simulink model "Pendulum"  (Simulink 5.0)
settings: Solver=ode45  StartTime=0.0  StopTime=inf  RelTol=1e-12  AbsTol=1e-9
values from neighbouring files (symbols this model uses):
  N = Nu + K*Nx    [PENDULUM.M]
libraries: mblibv1 x8
settings Model: LastModifiedBy=Administrator  BooleanDataType=off

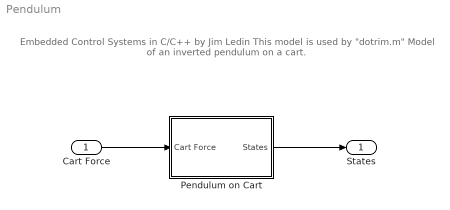
== system Pendulum ==
  note: Embedded Control Systems in C/C++
      | by Jim Ledin
      |
      | This model is used by "dotrim.m"
      |
      | Model of an inverted pendulum on a cart.
  Cart Force : Inport  PortDimensions=1
  Pendulum on Cart : Subsystem
  States : Outport
  wires:
  Cart Force/1 -> Pendulum on Cart/1(Cart Force)
  Pendulum on Cart/1(States) -> States/1

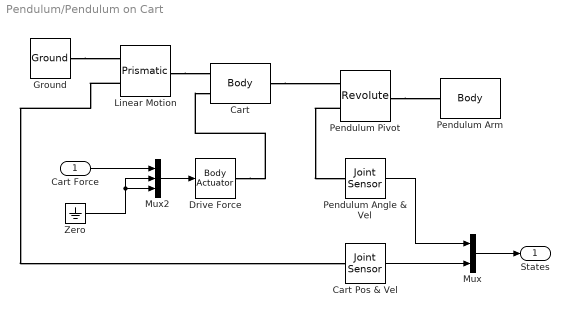
== system Pendulum/Pendulum on Cart ==
  Cart Force : Inport  PortDimensions=1
  Cart : mblibv1/Bodies/Body  Tag=Factory generic  Description=Mechanical Blockset  PhysicalDomain=mechanical  SubClassName=Unknown  PortType=workingframe  LConnTagsString=CS1|CG  RConnTagsString=CS2  DialogClass=MechanicalBodyBlock  Mass=5  MassUnits=kg  InertiaUnits=kg*m^2  Inertia=eye(3)  Shape=Cylinder  ShapeDims=[1 1]  ShapeUnits=m  ShapeUse=false  Density=1  DensityUnits=kg/m^3  DensityUse=false  CG=Left$CG$[0 0 0]$WORLD$WORLD$m$[0 0 0]$Euler X-Y-Z$deg$WORLD$true  WorkingFrames=Left$CS1$[0 0 0]$CG$CG$m$[0 0 0]$Euler X-Y-Z$deg$WORLD$true#Right$CS2$[0 0 0]$CG$CG$m$[0 0 0]$Euler X-Y-Z$deg$WORLD$true
  Cart Pos & Vel : mblibv1/Sensors &  Actuators/Joint Sensor  Tag=__orphan__  Description=Mechanical Blockset  PortType=blob  PhysicalDomain=Mechanical  Muxed=on  Pose=off  Angle=on  AngleUnits=deg  ArcVelocity=off  ArcVelocityUnits=deg/s  ArcAcceleration=off  ArcAccelerationUnits=deg/s²  CoordPosition=on  CoordPositionUnits=m  Velocity=on  VelocityUnits=m/s  Acceleration=off  AccelerationUnits=m/s²  Quaternion=on  QuaternionDT=off  QuaternionDDT=off  QuaternionUnits=off  OutputVector=[ 1 1 ]  ActiveIO=off  Width=1  DialogClass=MechanicalSensorBlock  Primitive=P1  Force=off  ForceUnits=N  Torque=off  TorqueUnits=N-m  ReferenceFrame=Absolute (INERTIAL)  ReactionSensedSide=Base  ReactionReferenceFrame=Absolute (World)  ReactionForce=off  ReactionForceUnits=N  ReactionMoment=off  ReactionMomentUnits=N-m
  Drive Force : mblibv1/Sensors &  Actuators/Body Actuator  Tag=__orphan__  Description=Mechanical Blockset  PortType=blob  PhysicalDomain=Mechanical  ActuationStyle=Force  AngleUnits=deg  ArcVelocityUnits=deg/s  ArcAccelerationUnits=deg/s^2  CoordPositionUnits=m  VelocityUnits=m/s  AccelerationUnits=m/s^2  ForceUnits=N  TorqueUnits=N-m  ActiveIO=off  Width=1  DialogClass=MechanicalActuatorBlock  ReferenceFrame=Absolute (INERTIAL)  Angle=off  CoordPosition=on  Force=on  Torque=off
  Ground : mblibv1/Bodies/Ground  Tag=__orphan__  PortType=workingframe  PhysicalDomain=Mechanical  DialogClass=GroundBlock  CoordPosition=[0 0 0]  CoordPositionUnits=m  StateVectorMgrId=-1  MachineId=[0 0]
  Linear Motion : mblibv1/Joints/Prismatic  Tag=Factory generic  Description=Mechanical Blockset  PhysicalDomain=mechanical  SubClassName=Unknown  PortType=blob  LConnTagsString=__newl0|SA1  RConnTagsString=__newr0  NumSAPorts=1  CutJoint=off  MarkAsCut=off  Primitives=prismatic  PrimitiveProps=P1$WORLD$[1 0 0]$prismatic  DialogClass=JointBlock
  Mux : Mux  Inputs=2
  Mux2 : Mux  Inputs=3
  Pendulum Angle & Vel : mblibv1/Sensors &  Actuators/Joint Sensor  Tag=__orphan__  Description=Mechanical Blockset  PortType=blob  PhysicalDomain=Mechanical  Muxed=on  Pose=off  Angle=on  AngleUnits=rad  ArcVelocity=on  ArcVelocityUnits=rad/s  ArcAcceleration=off  ArcAccelerationUnits=deg/s^2  CoordPosition=on  CoordPositionUnits=m  Velocity=off  VelocityUnits=m/s  Acceleration=off  AccelerationUnits=m/s^2  Quaternion=on  QuaternionDT=off  QuaternionDDT=off  QuaternionUnits=off  OutputVector=[ 1 1 ]  ActiveIO=off  Width=1  DialogClass=MechanicalSensorBlock  Primitive=R1  Force=off  ForceUnits=N  Torque=off  TorqueUnits=N-m  ReferenceFrame=Absolute (INERTIAL)  ReactionSensedSide=Base  ReactionReferenceFrame=Absolute (World)  ReactionForce=off  ReactionForceUnits=N  ReactionMoment=off  ReactionMomentUnits=N-m
  Pendulum Arm : mblibv1/Bodies/Body  Tag=Factory generic  Description=Mechanical Blockset  PhysicalDomain=mechanical  SubClassName=Unknown  PortType=workingframe  LConnTagsString=CS1  DialogClass=MechanicalBodyBlock  Mass=2.49  MassUnits=kg  InertiaUnits=kg*m^2  Inertia=[1.25e-4 0 0; 0 .208 0; 0 0 .208]  Shape=Cylinder  ShapeDims=[1 1]  ShapeUnits=m  ShapeUse=false  Density=1  DensityUnits=kg/m^3  DensityUse=false  CG=Left$CG$[0 .5 0]$WORLD$WORLD$m$[0 0 0]$Euler X-Y-Z$deg$WORLD$false  WorkingFrames=Left$CS1$[0 0 0]$WORLD$WORLD$m$[0 0 0]$Euler X-Y-Z$deg$WORLD$true#Right$CS2$[0 0 0]$CG$CG$m$[0 0 0]$Euler X-Y-Z$deg$WORLD$false
  Pendulum Pivot : mblibv1/Joints/Revolute  Tag=Factory generic  Description=Mechanical Blockset  PhysicalDomain=mechanical  SubClassName=Unknown  PortType=blob  LConnTagsString=__newl0|SA1  RConnTagsString=__newr0  NumSAPorts=1  CutJoint=off  MarkAsCut=off  Primitives=revolute  PrimitiveProps=R1$WORLD$[0 0 -1]$revolute  DialogClass=JointBlock
  Zero : Ground
  States : Outport
  wires:
  Pendulum Angle & Vel/1 -> Mux/1
  Cart Pos & Vel/1 -> Mux/2
  Mux/1 -> States/1
  Mux2/1 -> Drive Force/1
  Zero/1 -> Mux2/2, Mux2/3
  Cart Force/1 -> Mux2/1
  connections:
  Pendulum Pivot/RConn1 -- Pendulum Arm/LConn1
  Ground/RConn1 -- Linear Motion/LConn1
  Cart/RConn1 -- Pendulum Pivot/LConn1
  Linear Motion/RConn1 -- Cart/LConn1
  Pendulum Pivot/LConn2 -- Pendulum Angle & Vel/LConn1
  Linear Motion/LConn2 -- Cart Pos & Vel/LConn1
  Drive Force/RConn1 -- Cart/LConn2
